simulink model "SiEnginePx"  (R2021b)
settings: Solver=VariableStepAuto  StartTime=0.0  StopTime=inf  RelTol=1e-3  EnableMultiTasking=on
InitFcn:
  | autoicon('autolibsiengcal',gcs,'varSwitched');
model workspace (MAT data in the model file):
  AccPwrbp = [0 0]
  AccSpdbp = [300 750]
  AfrStoich = 14.6
  TimeCnstECP = 0.125
  TimeCnstEGR = 0.125
  TimeCnstETC = 0.085
  TimeCnstICP = 0.125
  TimeCnstIVL = 0.125
  TimeCnstSWVA = 0.125
  TimeCnstVCR = 0.125
  TimeCnstVGT = 0.15
  TimeCnstVIRL = 0.125
  TimeCnstWGA = 0.15
  f_twc_eff_co = [0.17 0.25 0.45 0.99 0.99 0.99 0.99]
  f_twc_eff_hc = [0.21 0.375 0.75 0.98 0.98 0.98 0.98]
  f_twc_eff_lam = [0.909090909 0.944055944 0.979020979 1 1.013986014 1.048951049 1.083916084]
  f_twc_eff_nox = [0.98 0.98 0.98 0.97 0.05 0.02 0]
libraries: autolibhevctrlrcommon x1, autolibpowerinfoutils x1, autolibutils x1
settings Model: DataDictionary=SiEnginePx.sldd  ModifiedByFormat=The MathWorks, Inc.  SimulationMode=accelerator  Creator=The MathWorks, Inc.  LastModifiedBy=The MathWorks, Inc.
settings SolverCC: AlgebraicLoopSolver=TrustRegion  DecoupledContinuousIntegration=on
settings DataIOCC: DSMLogging=off  ReturnWorkspaceOutputs=off
settings DebuggingCC: ModelReferenceExtraNoncontSigs=none  SFMachineParentedDataDiag=warning  ArithmeticOperatorsInVariantConditions=warning
settings SFSimCC: SimUseLocalCustomCode=off  CustomCodeUndefinedFunction=UseInterfaceOnly
settings RTWCC: RTWUseLocalCustomCode=off
settings CodeAppCC: StateflowObjectComments=on
settings GRTTargetCC: TargetLangStandard=C89/C90 (ANSI)
settings ConfigComp: CovMetricSettings=dsw  CovSaveCumulativeToWorkspaceVar=on  CovSaveSingleToWorkspaceVar=on  CovExternalEMLEnable=off
settings SimscapeCC: SimscapeNormalizeSystem=off  SimscapeNominalValues={1, 'bar'; 1, 'cm^3/s'; 1, 'bar*kg/s'; 1, 'kJ/kg'; 1, 'kW'; };

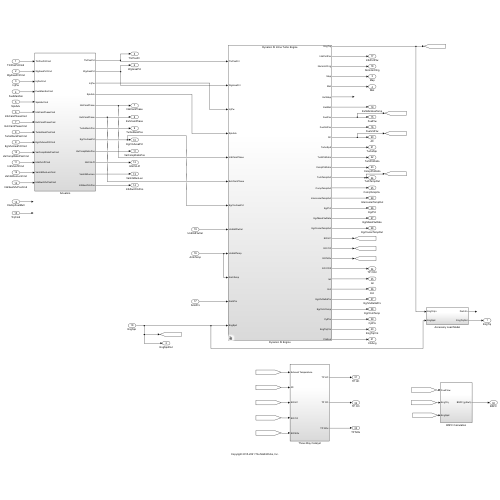
[thumbnail: Simulink's stored preview of the top-level diagram]
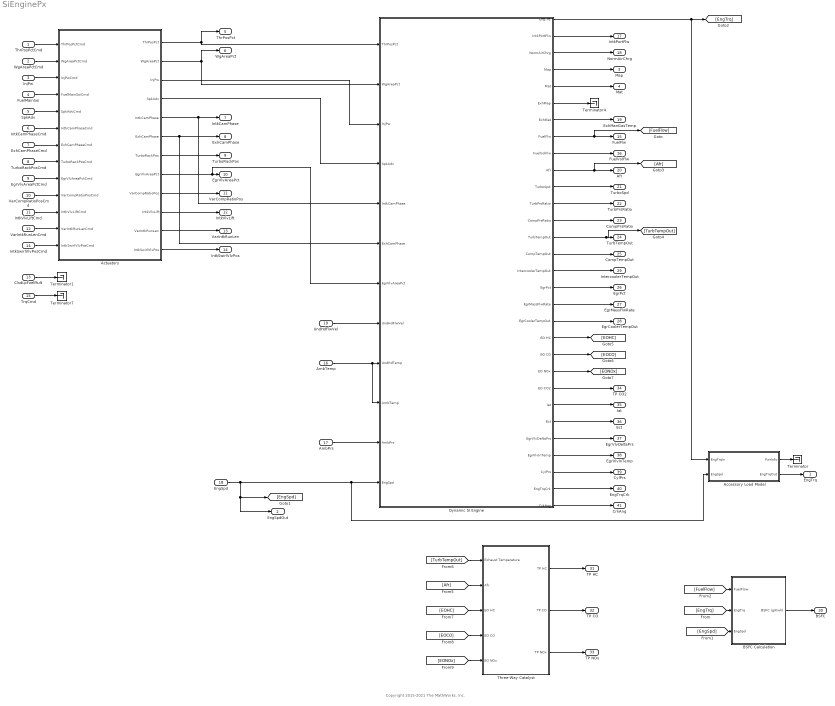
== system SiEnginePx ==
  note: Copyright 2015-2021 The MathWorks, Inc.
  ThrPosPctCmd : Inport
  WgAreaPctCmd : Inport  Port=2
  InjPw : Inport  Port=3
  FuelMainSoi : Inport  Port=4
  SpkAdv : Inport  Port=5
  IntkCamPhaseCmd : Inport  Port=6
  ExhCamPhaseCmd : Inport  Port=7
  TurboRackPosCmd : Inport  Port=8
  EgrVlvAreaPctCmd : Inport  Port=9
  VarCompRatioPosCmd : Inport  Port=10
  IntkVlvLiftCmd : Inport  Port=11
  VarIntkRunLenCmd : Inport  Port=12
  ClsdLpFuelMult : Inport  Port=13  Unit=1
  IntkSwirlVlvPosCmd : Inport  Port=14
  TrqCmd : Inport  Port=15  Unit=N*m
  AmbTemp : Inport  Port=16
  AmbPrs : Inport  Port=17
  EngSpd : Inport  Port=18  Interpolate=off
  UndHdFlwVel : Inport  Port=19
  Accessory Load Model : Subsystem
  Actuators : Subsystem
  BSFC Calculation : Subsystem
  Dynamic SI Engine : Subsystem  Variant=on  VariantControlMode=label  VariantControl=Choice  LabelModeActiveChoice=SiEngineCore
  Terminator{,1,4,7} (4 alike) : Terminator
  Three-Way Catalyst : Subsystem
  EngTrq : Outport  Unit=N*m  VectorParamsAs1DForOutWhenUnconnected=off
  EngSpdOut : Outport  Port=2  VectorParamsAs1DForOutWhenUnconnected=off
  Map : Outport  Port=3  VectorParamsAs1DForOutWhenUnconnected=off
  Mat : Outport  Port=4  VectorParamsAs1DForOutWhenUnconnected=off
  ThrPosPct : Outport  Port=5  VectorParamsAs1DForOutWhenUnconnected=off
  WgAreaPct : Outport  Port=6  VectorParamsAs1DForOutWhenUnconnected=off
  IntkCamPhase : Outport  Port=7  VectorParamsAs1DForOutWhenUnconnected=off
  ExhCamPhase : Outport  Port=8  VectorParamsAs1DForOutWhenUnconnected=off
  TurboRackPos : Outport  Port=9  VectorParamsAs1DForOutWhenUnconnected=off
  EgrVlvAreaPct : Outport  Port=10  VectorParamsAs1DForOutWhenUnconnected=off
  VarCompRatioPos : Outport  Port=11  VectorParamsAs1DForOutWhenUnconnected=off
  IntkVlvLift : Outport  Port=12  VectorParamsAs1DForOutWhenUnconnected=off
  VarIntkRunLen : Outport  Port=13  VectorParamsAs1DForOutWhenUnconnected=off
  IntkSwirlVlvPos : Outport  Port=14  VectorParamsAs1DForOutWhenUnconnected=off
  FuelFlw : Outport  Port=15  VectorParamsAs1DForOutWhenUnconnected=off
  FuelVolFlw : Outport  Port=16  VectorParamsAs1DForOutWhenUnconnected=off
  IntkPortFlw : Outport  Port=17  VectorParamsAs1DForOutWhenUnconnected=off
  NormAirChrg : Outport  Port=18  VectorParamsAs1DForOutWhenUnconnected=off
  ExhManGasTemp : Outport  Port=19  VectorParamsAs1DForOutWhenUnconnected=off
  Afr : Outport  Port=20  VectorParamsAs1DForOutWhenUnconnected=off
  TurboSpd : Outport  Port=21  VectorParamsAs1DForOutWhenUnconnected=off
  TurbPrsRatio : Outport  Port=22  VectorParamsAs1DForOutWhenUnconnected=off
  CompPrsRatio : Outport  Port=23  VectorParamsAs1DForOutWhenUnconnected=off
  TurbTempOut : Outport  Port=24  VectorParamsAs1DForOutWhenUnconnected=off
  CompTempOut : Outport  Port=25  VectorParamsAs1DForOutWhenUnconnected=off
  EgrPct : Outport  Port=26  Unit=%  VectorParamsAs1DForOutWhenUnconnected=off
  EgrMassFlwRate : Outport  Port=27  Unit=kg/s  VectorParamsAs1DForOutWhenUnconnected=off
  EgrCoolerTempOut : Outport  Port=28  Unit=K  VectorParamsAs1DForOutWhenUnconnected=off
  IntercoolerTempOut : Outport  Port=29  VectorParamsAs1DForOutWhenUnconnected=off
  BSFC : Outport  Port=30  Unit=g/(kW*hr)  VectorParamsAs1DForOutWhenUnconnected=off
  TP HC : Outport  Port=31  VectorParamsAs1DForOutWhenUnconnected=off
  TP CO : Outport  Port=32  VectorParamsAs1DForOutWhenUnconnected=off
  TP NOx : Outport  Port=33  VectorParamsAs1DForOutWhenUnconnected=off
  TP CO2 : Outport  Port=34  VectorParamsAs1DForOutWhenUnconnected=off
  Iat : Outport  Port=35  VectorParamsAs1DForOutWhenUnconnected=off
  Ect : Outport  Port=36  VectorParamsAs1DForOutWhenUnconnected=off
  EgrVlvDeltaPrs : Outport  Port=37  VectorParamsAs1DForOutWhenUnconnected=off
  EgrVlvInTemp : Outport  Port=38  VectorParamsAs1DForOutWhenUnconnected=off
  CylPrs : Outport  Port=39  VectorParamsAs1DForOutWhenUnconnected=off
  EngTrqCrk : Outport  Port=40  VectorParamsAs1DForOutWhenUnconnected=off
  CrkAng : Outport  Port=41  VectorParamsAs1DForOutWhenUnconnected=off
  wires:
  SpkAdv/1 -> Actuators/5(SpkAdvCmd)
  InjPw/1 -> Actuators/3(InjPwCmd)
  EngSpd/1 -> EngSpdOut/1, [EngSpd], Dynamic SI Engine/12(EngSpd), Accessory Load Model/2(EngSpd)
  [FuelFlow] -> BSFC Calculation/1(FuelFlow)
  [EngTrq] -> BSFC Calculation/2(EngTrq)
  [EngSpd] -> BSFC Calculation/3(EngSpd)
  BSFC Calculation/1(BSFC (g/Kwh)) -> BSFC/1
  Three-Way Catalyst/1(TP HC) -> TP HC/1
  Three-Way Catalyst/2(TP CO) -> TP CO/1
  Three-Way Catalyst/3(TP NOx) -> TP NOx/1
  [TurbTempOut] -> Three-Way Catalyst/1(Exhaust Temperature)
  [Afr] -> Three-Way Catalyst/2(Afr)
  ThrPosPctCmd/1 -> Actuators/1(ThrPosPctCmd)
  WgAreaPctCmd/1 -> Actuators/2(WgAreaPctCmd)
  IntkCamPhaseCmd/1 -> Actuators/6(IntkCamPhaseCmd)
  ExhCamPhaseCmd/1 -> Actuators/7(ExhCamPhaseCmd)
  TrqCmd/1 -> Terminator7/1
  [EOHC] -> Three-Way Catalyst/3(EO HC)
  [EOCO] -> Three-Way Catalyst/4(EO CO)
  [EONOx] -> Three-Way Catalyst/5(EO NOx)
  Actuators/1(ThrPosPct) -> ThrPosPct/1, Dynamic SI Engine/1(ThrPosPct)
  Actuators/2(WgAreaPct) -> WgAreaPct/1, Dynamic SI Engine/2(WgAreaPct)
  Actuators/5(IntkCamPhase) -> IntkCamPhase/1, Dynamic SI Engine/5(IntkCamPhase)
  Actuators/6(ExhCamPhase) -> ExhCamPhase/1, Dynamic SI Engine/6(ExhCamPhase)
  FuelMainSoi/1 -> Actuators/4(FuelMainSoiCmd)
  TurboRackPosCmd/1 -> Actuators/8(TurboRackPosCmd)
  EgrVlvAreaPctCmd/1 -> Actuators/9(EgrVlvAreaPctCmd)
  VarCompRatioPosCmd/1 -> Actuators/10(VarCompRatioPosCmd)
  IntkVlvLiftCmd/1 -> Actuators/11(IntkVlvLiftCmd)
  VarIntkRunLenCmd/1 -> Actuators/12(VarIntkRunLenCmd)
  IntkSwirlVlvPosCmd/1 -> Actuators/13(IntkSwirlVlvPosCmd)
  Actuators/7(TurboRackPos) -> TurboRackPos/1
  Actuators/8(EgrVlvAreaPct) -> EgrVlvAreaPct/1, Dynamic SI Engine/7(EgrVlvAreaPct)
  Actuators/9(VarCompRatioPos) -> VarCompRatioPos/1
  Actuators/10(IntkVlvLift) -> IntkVlvLift/1
  Actuators/11(VarIntkRunLen) -> VarIntkRunLen/1
  Actuators/12(IntkSwirlVlvPos) -> IntkSwirlVlvPos/1
  Accessory Load Model/2(EngTrqOut) -> EngTrq/1
  Accessory Load Model/1(PwrInfo) -> Terminator/1
  ClsdLpFuelMult/1 -> Terminator1/1
  Actuators/3(InjPw) -> Dynamic SI Engine/3(InjPw)
  Actuators/4(SpkAdv) -> Dynamic SI Engine/4(SpkAdv)
  UndHdFlwVel/1 -> Dynamic SI Engine/8(UndHdFlwVel)
  AmbTemp/1 -> Dynamic SI Engine/9(UndHdTemp), Dynamic SI Engine/10(AmbTemp)
  AmbPrs/1 -> Dynamic SI Engine/11(AmbPrs)
  Dynamic SI Engine/1(EngTrq) -> [EngTrq], Accessory Load Model/1(EngTrqIn)
  Dynamic SI Engine/2(IntkPortFlw) -> IntkPortFlw/1
  Dynamic SI Engine/3(NormAirChrg) -> NormAirChrg/1
  Dynamic SI Engine/4(Map) -> Map/1
  Dynamic SI Engine/5(Mat) -> Mat/1
  Dynamic SI Engine/6(ExhMap) -> Terminator4/1
  Dynamic SI Engine/7(ExhMat) -> ExhManGasTemp/1
  Dynamic SI Engine/8(FuelFlw) -> FuelFlw/1, [FuelFlow]
  Dynamic SI Engine/9(FuelVolFlw) -> FuelVolFlw/1
  Dynamic SI Engine/10(Afr) -> Afr/1, [Afr]
  Dynamic SI Engine/11(TurboSpd) -> TurboSpd/1
  Dynamic SI Engine/12(TurbPrsRatio) -> TurbPrsRatio/1
  Dynamic SI Engine/13(CompPrsRatio) -> CompPrsRatio/1
  Dynamic SI Engine/14(TurbTempOut) -> [TurbTempOut], TurbTempOut/1
  Dynamic SI Engine/15(CompTempOut) -> CompTempOut/1
  Dynamic SI Engine/16(IntercoolerTempOut) -> IntercoolerTempOut/1
  Dynamic SI Engine/17(EgrPct) -> EgrPct/1
  Dynamic SI Engine/18(EgrMassFlwRate) -> EgrMassFlwRate/1
  Dynamic SI Engine/19(EgrCoolerTempOut) -> EgrCoolerTempOut/1
  Dynamic SI Engine/20(EO HC) -> [EOHC]
  Dynamic SI Engine/21(EO CO) -> [EOCO]
  Dynamic SI Engine/22(EO NOx) -> [EONOx]
  Dynamic SI Engine/23(EO CO2) -> TP CO2/1
  Dynamic SI Engine/24(Iat) -> Iat/1
  Dynamic SI Engine/25(Ect) -> Ect/1
  Dynamic SI Engine/26(EgrVlvDeltaPrs) -> EgrVlvDeltaPrs/1
  Dynamic SI Engine/27(EgrVlvInTemp) -> EgrVlvInTemp/1
  Dynamic SI Engine/28(CylPrs) -> CylPrs/1
  Dynamic SI Engine/29(EngTrqCrk) -> EngTrqCrk/1
  Dynamic SI Engine/30(CrkAng) -> CrkAng/1

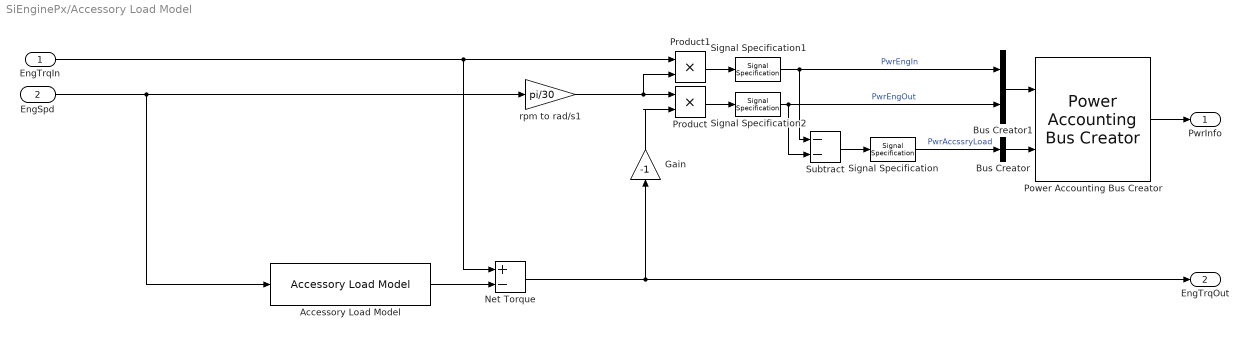
== system SiEnginePx/Accessory Load Model ==
  EngTrqIn : Inport
  EngSpd : Inport  Port=2
  Accessory Load Model : autolibhevctrlrcommon/Accessory Load Model  AccPwrTbl=[0 0]  AccSpdBpts=[300 750]
      settings: SourceProductBaseCode=PW
  Bus Creator : BusCreator  Inputs=1
  Bus Creator1 : BusCreator  Inputs=2
  Gain : Gain  Gain=-1
  Net Torque : Sum  Inputs=+-
  Power Accounting Bus Creator : autolibpowerinfoutils/Power Accounting Bus Creator  AssctBlkSelPopup=Parent  RefBlkName='libraryname/blkname'  PwrTrnsfrdCheckBox=on  PwrNotTrnsfrdCheckBox=on  PwrStoredCheckBox=off  aMode=aMode
      settings: SourceProductBaseCode=PW,DR,MT,UV,VE
  Product : Product
  Product1 : Product
  Signal Specification : SignalSpecification  Unit=W
  Signal Specification1 : SignalSpecification  Unit=W
  Signal Specification2 : SignalSpecification  Unit=W
  Subtract : Sum  Inputs=--
  rpm to rad/s1 : Gain  Gain=pi/30
  PwrInfo : Outport  VectorParamsAs1DForOutWhenUnconnected=off
  EngTrqOut : Outport  Port=2  Unit=N*m  VectorParamsAs1DForOutWhenUnconnected=off
  wires:
  Accessory Load Model/1 -> Net Torque/2
  EngSpd/1 -> Accessory Load Model/1, rpm to rad/s1/1
  Net Torque/1 -> EngTrqOut/1, Gain/1
  Bus Creator/1 -> Power Accounting Bus Creator/2
  Bus Creator1/1 -> Power Accounting Bus Creator/1
  EngTrqIn/1 -> Product1/1, Net Torque/1
  Subtract/1 -> Signal Specification/1
  Signal Specification/1 -> Bus Creator/1  "PwrAccssryLoad"
  Power Accounting Bus Creator/1 -> PwrInfo/1
  Product/1 -> Signal Specification2/1
  Product1/1 -> Signal Specification1/1
  rpm to rad/s1/1 -> Product1/2, Product/1
  Signal Specification1/1 -> Subtract/1, Bus Creator1/1  "PwrEngIn"
  Signal Specification2/1 -> Subtract/2, Bus Creator1/2  "PwrEngOut"
  Gain/1 -> Product/2

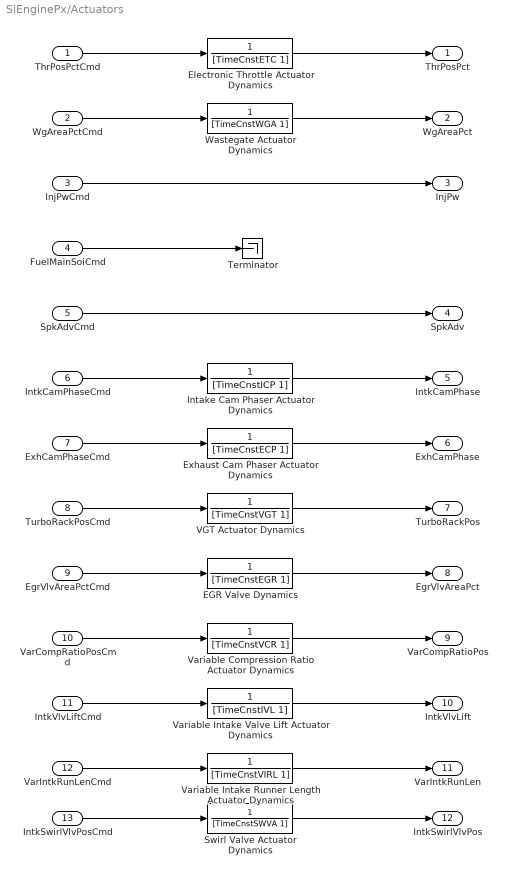
== system SiEnginePx/Actuators ==
  ThrPosPctCmd : Inport  Unit=%
  WgAreaPctCmd : Inport  Port=2  Unit=%
  InjPwCmd : Inport  Port=3  Unit=ms
  FuelMainSoiCmd : Inport  Port=4  Unit=deg
  SpkAdvCmd : Inport  Port=5  Unit=deg
  IntkCamPhaseCmd : Inport  Port=6  Unit=deg
  ExhCamPhaseCmd : Inport  Port=7  Unit=deg
  TurboRackPosCmd : Inport  Port=8  Unit=1
  EgrVlvAreaPctCmd : Inport  Port=9  Unit=%
  VarCompRatioPosCmd : Inport  Port=10
  IntkVlvLiftCmd : Inport  Port=11
  VarIntkRunLenCmd : Inport  Port=12
  IntkSwirlVlvPosCmd : Inport  Port=13
  EGR Valve Dynamics : TransferFcn  Denominator=[TimeCnstEGR 1]
  Electronic Throttle Actuator Dynamics : TransferFcn  Denominator=[TimeCnstETC 1]
  Exhaust Cam Phaser Actuator Dynamics : TransferFcn  Denominator=[TimeCnstECP 1]
  Intake Cam Phaser Actuator Dynamics : TransferFcn  Denominator=[TimeCnstICP 1]
  Swirl Valve Actuator Dynamics : TransferFcn  Denominator=[TimeCnstSWVA 1]
  Terminator : Terminator
  VGT Actuator Dynamics : TransferFcn  Denominator=[TimeCnstVGT 1]
  Variable Compression Ratio Actuator Dynamics : TransferFcn  Denominator=[TimeCnstVCR 1]
  Variable Intake Runner Length Actuator Dynamics : TransferFcn  Denominator=[TimeCnstVIRL 1]
  Variable Intake Valve Lift Actuator Dynamics : TransferFcn  Denominator=[TimeCnstIVL 1]
  Wastegate Actuator Dynamics : TransferFcn  Denominator=[TimeCnstWGA 1]
  ThrPosPct : Outport  Unit=%  VectorParamsAs1DForOutWhenUnconnected=off
  WgAreaPct : Outport  Port=2  Unit=%  VectorParamsAs1DForOutWhenUnconnected=off
  InjPw : Outport  Port=3  VectorParamsAs1DForOutWhenUnconnected=off
  SpkAdv : Outport  Port=4  VectorParamsAs1DForOutWhenUnconnected=off
  IntkCamPhase : Outport  Port=5  Unit=deg  VectorParamsAs1DForOutWhenUnconnected=off
  ExhCamPhase : Outport  Port=6  Unit=deg  VectorParamsAs1DForOutWhenUnconnected=off
  TurboRackPos : Outport  Port=7  Unit=1  VectorParamsAs1DForOutWhenUnconnected=off
  EgrVlvAreaPct : Outport  Port=8  Unit=%  VectorParamsAs1DForOutWhenUnconnected=off
  VarCompRatioPos : Outport  Port=9  VectorParamsAs1DForOutWhenUnconnected=off
  IntkVlvLift : Outport  Port=10  VectorParamsAs1DForOutWhenUnconnected=off
  VarIntkRunLen : Outport  Port=11  VectorParamsAs1DForOutWhenUnconnected=off
  IntkSwirlVlvPos : Outport  Port=12  VectorParamsAs1DForOutWhenUnconnected=off
  wires:
  Variable Compression Ratio Actuator Dynamics/1 -> VarCompRatioPos/1
  Variable Intake Valve Lift Actuator Dynamics/1 -> IntkVlvLift/1
  Variable Intake Runner Length Actuator Dynamics/1 -> VarIntkRunLen/1
  Swirl Valve Actuator Dynamics/1 -> IntkSwirlVlvPos/1
  Intake Cam Phaser Actuator Dynamics/1 -> IntkCamPhase/1
  Exhaust Cam Phaser Actuator Dynamics/1 -> ExhCamPhase/1
  Wastegate Actuator Dynamics/1 -> WgAreaPct/1
  Electronic Throttle Actuator Dynamics/1 -> ThrPosPct/1
  FuelMainSoiCmd/1 -> Terminator/1
  IntkVlvLiftCmd/1 -> Variable Intake Valve Lift Actuator Dynamics/1
  IntkSwirlVlvPosCmd/1 -> Swirl Valve Actuator Dynamics/1
  WgAreaPctCmd/1 -> Wastegate Actuator Dynamics/1
  ThrPosPctCmd/1 -> Electronic Throttle Actuator Dynamics/1
  ExhCamPhaseCmd/1 -> Exhaust Cam Phaser Actuator Dynamics/1
  IntkCamPhaseCmd/1 -> Intake Cam Phaser Actuator Dynamics/1
  VarCompRatioPosCmd/1 -> Variable Compression Ratio Actuator Dynamics/1
  VarIntkRunLenCmd/1 -> Variable Intake Runner Length Actuator Dynamics/1
  InjPwCmd/1 -> InjPw/1
  VGT Actuator Dynamics/1 -> TurboRackPos/1
  EGR Valve Dynamics/1 -> EgrVlvAreaPct/1
  TurboRackPosCmd/1 -> VGT Actuator Dynamics/1
  EgrVlvAreaPctCmd/1 -> EGR Valve Dynamics/1
  SpkAdvCmd/1 -> SpkAdv/1

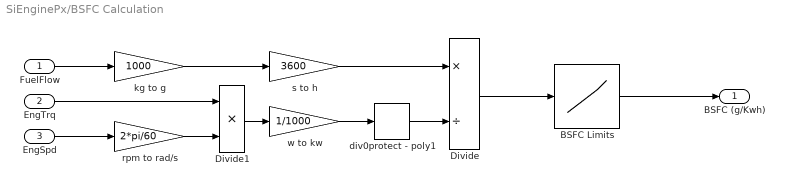
== system SiEnginePx/BSFC Calculation ==
  FuelFlow : Inport
  EngTrq : Inport  Port=2
  EngSpd : Inport  Port=3
  BSFC Limits : Lookup_n-D  NumberOfTableDimensions=1  BreakpointsForDimension1=[0 500]  Table=[0 500]  ExtrapMethod=Clip  InternalRulePriority=Speed  RndMeth=Simplest  InputSameDT=on
  Divide : Product  Inputs=*/
  Divide1 : Product  Inputs=**
  div0protect - poly1 : autolibutils/div0protect - poly  thresh=1e-6  ZeroCross1=off  aMode=aMode
      settings: SourceProductBaseCode=PW,DR,MT,UV,VE
  kg to g : Gain  Gain=1000
  rpm to rad/s : Gain  Gain=2*pi/60
  s to h : Gain  Gain=3600
  w to kw : Gain  Gain=1/1000
  BSFC (g/Kwh) : Outport  VectorParamsAs1DForOutWhenUnconnected=off
  wires:
  Divide1/1 -> w to kw/1
  kg to g/1 -> s to h/1
  FuelFlow/1 -> kg to g/1
  rpm to rad/s/1 -> Divide1/2
  EngSpd/1 -> rpm to rad/s/1
  EngTrq/1 -> Divide1/1
  Divide/1 -> BSFC Limits/1
  w to kw/1 -> div0protect - poly1/1
  s to h/1 -> Divide/1
  BSFC Limits/1 -> BSFC (g/Kwh)/1
  div0protect - poly1/1 -> Divide/2

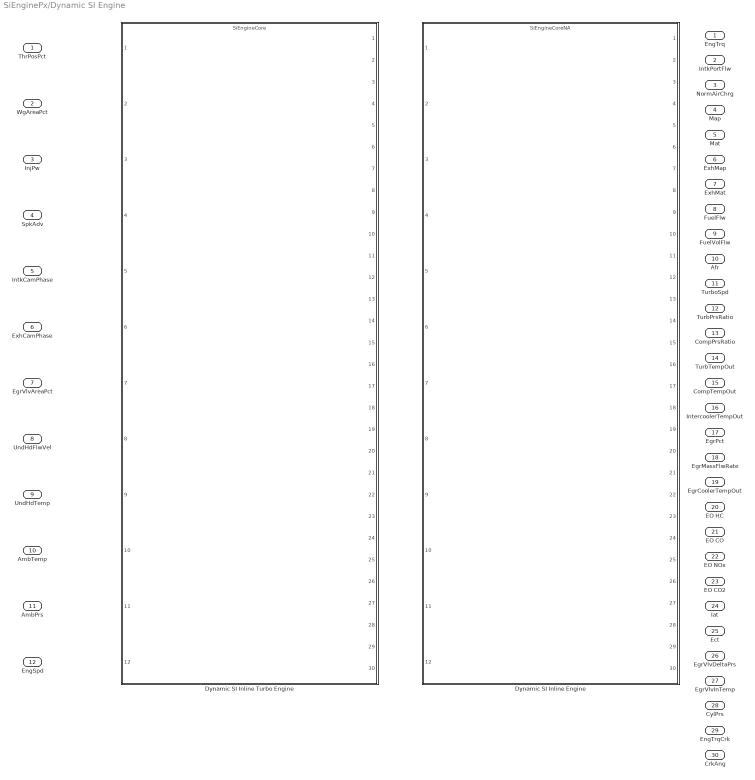
== system SiEnginePx/Dynamic SI Engine ==
  ThrPosPct : Inport
  WgAreaPct : Inport  Port=2
  InjPw : Inport  Port=3
  SpkAdv : Inport  Port=4
  IntkCamPhase : Inport  Port=5
  ExhCamPhase : Inport  Port=6
  EgrVlvAreaPct : Inport  Port=7
  UndHdFlwVel : Inport  Port=8
  UndHdTemp : Inport  Port=9
  AmbTemp : Inport  Port=10
  AmbPrs : Inport  Port=11
  EngSpd : Inport  Port=12
  Dynamic SI Inline Engine : ModelReference  ModelNameDialog=SiEngineCoreNA.slx  SimulationMode=Normal  VariantControl=SiEngineCoreNA  ModelReferenceVersion=3.4
  Dynamic SI Inline Turbo Engine : ModelReference  ModelNameDialog=SiEngineCore.slx  SimulationMode=Normal  VariantControl=SiEngineCore  ModelReferenceVersion=3.4
  EngTrq : Outport
  IntkPortFlw : Outport  Port=2
  NormAirChrg : Outport  Port=3
  Map : Outport  Port=4
  Mat : Outport  Port=5
  ExhMap : Outport  Port=6
  ExhMat : Outport  Port=7
  FuelFlw : Outport  Port=8
  FuelVolFlw : Outport  Port=9
  Afr : Outport  Port=10
  TurboSpd : Outport  Port=11
  TurbPrsRatio : Outport  Port=12
  CompPrsRatio : Outport  Port=13
  TurbTempOut : Outport  Port=14
  CompTempOut : Outport  Port=15
  IntercoolerTempOut : Outport  Port=16
  EgrPct : Outport  Port=17
  EgrMassFlwRate : Outport  Port=18
  EgrCoolerTempOut : Outport  Port=19
  EO HC : Outport  Port=20
  EO CO : Outport  Port=21
  EO NOx : Outport  Port=22
  EO CO2 : Outport  Port=23
  Iat : Outport  Port=24
  Ect : Outport  Port=25
  EgrVlvDeltaPrs : Outport  Port=26
  EgrVlvInTemp : Outport  Port=27
  CylPrs : Outport  Port=28  VectorParamsAs1DForOutWhenUnconnected=off
  EngTrqCrk : Outport  Port=29  VectorParamsAs1DForOutWhenUnconnected=off
  CrkAng : Outport  Port=30  VectorParamsAs1DForOutWhenUnconnected=off

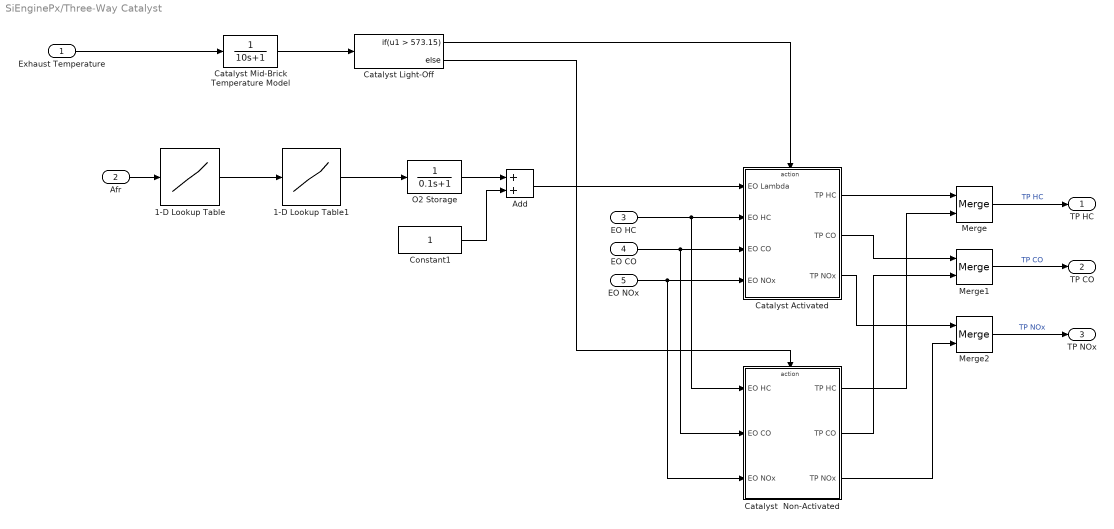
== system SiEnginePx/Three-Way Catalyst ==
  Exhaust Temperature : Inport
  Afr : Inport  Port=2
  EO HC : Inport  Port=3
  EO CO : Inport  Port=4
  EO NOx : Inport  Port=5
  1-D Lookup Table : Lookup_n-D  NumberOfTableDimensions=1  BreakpointsForDimension1=[0 15 100]  Table=[0 15 AfrStoich]/AfrStoich  ExtrapMethod=Clip  InternalRulePriority=Speed  RndMeth=Simplest  InputSameDT=on
  1-D Lookup Table1 : Lookup_n-D  NumberOfTableDimensions=1  BreakpointsForDimension1=[0 0.97 1.03 1.1]  Table=[-1 0 0 0.07]  ExtrapMethod=Clip  InternalRulePriority=Speed  RndMeth=Simplest  InputSameDT=on
  Add : Sum
  Catalyst  Non-Activated : Subsystem
  Catalyst Activated : Subsystem
  Catalyst Light-Off : If  IfExpression=u1 > 573.15
  "Catalyst Mid-Brick Temperature Model " : TransferFcn  Denominator=[10 1]
  Constant1 : Constant
  Merge : Merge
  Merge1 : Merge
  Merge2 : Merge
  O2 Storage : TransferFcn  Denominator=[0.1 1]
  TP HC : Outport  Unit=kg/s  VectorParamsAs1DForOutWhenUnconnected=off
  TP CO : Outport  Port=2  Unit=kg/s  VectorParamsAs1DForOutWhenUnconnected=off
  TP NOx : Outport  Port=3  Unit=kg/s  VectorParamsAs1DForOutWhenUnconnected=off
  wires:
  EO HC/1 -> Catalyst  Non-Activated/1(EO HC), Catalyst Activated/2(EO HC)
  EO CO/1 -> Catalyst  Non-Activated/2(EO CO), Catalyst Activated/3(EO CO)
  EO NOx/1 -> Catalyst  Non-Activated/3(EO NOx), Catalyst Activated/4(EO NOx)
  Merge/1 -> TP HC/1  "TP HC"
  Merge1/1 -> TP CO/1  "TP CO"
  Merge2/1 -> TP NOx/1  "TP NOx"
  Exhaust Temperature/1 -> "Catalyst Mid-Brick Temperature Model "/1
  Catalyst Light-Off/1 -> Catalyst Activated/Action
  Catalyst Light-Off/2 -> Catalyst  Non-Activated/Action
  "Catalyst Mid-Brick Temperature Model "/1 -> Catalyst Light-Off/1
  Catalyst Activated/1(TP HC) -> Merge/1
  Catalyst  Non-Activated/1(TP HC) -> Merge/2
  Catalyst Activated/2(TP CO) -> Merge1/1
  Catalyst  Non-Activated/2(TP CO) -> Merge1/2
  Catalyst Activated/3(TP NOx) -> Merge2/1
  Catalyst  Non-Activated/3(TP NOx) -> Merge2/2
  Add/1 -> Catalyst Activated/1(EO Lambda)
  1-D Lookup Table1/1 -> O2 Storage/1
  Constant1/1 -> Add/2
  O2 Storage/1 -> Add/1
  Afr/1 -> 1-D Lookup Table/1
  1-D Lookup Table/1 -> 1-D Lookup Table1/1

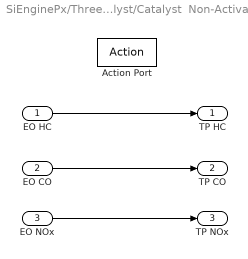
== system SiEnginePx/Three-Way Catalyst/Catalyst  Non-Activated ==
  EO HC : Inport
  EO CO : Inport  Port=2
  EO NOx : Inport  Port=3
  Action Port : ActionPort  ActionPortLabel=else
  TP HC : Outport  VectorParamsAs1DForOutWhenUnconnected=off
  TP CO : Outport  Port=2  VectorParamsAs1DForOutWhenUnconnected=off
  TP NOx : Outport  Port=3  VectorParamsAs1DForOutWhenUnconnected=off
  wires:
  EO HC/1 -> TP HC/1
  EO CO/1 -> TP CO/1
  EO NOx/1 -> TP NOx/1

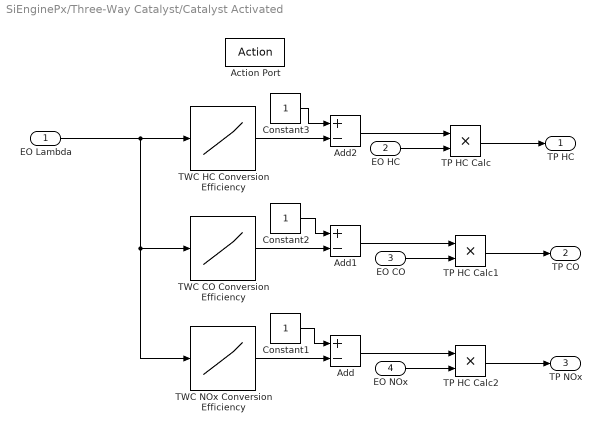
== system SiEnginePx/Three-Way Catalyst/Catalyst Activated ==
  EO Lambda : Inport
  EO HC : Inport  Port=2
  EO CO : Inport  Port=3
  EO NOx : Inport  Port=4
  Action Port : ActionPort  ActionPortLabel=if(u1 > 573.15)
  Add : Sum  Inputs=+-
  Add1 : Sum  Inputs=+-
  Add2 : Sum  Inputs=+-
  Constant1 : Constant
  Constant2 : Constant
  Constant3 : Constant
  TP HC Calc : Product  Inputs=**
  TP HC Calc1 : Product  Inputs=**
  TP HC Calc2 : Product  Inputs=**
  TWC CO Conversion Efficiency : Lookup_n-D  NumberOfTableDimensions=1  LookupTableObject=''  BreakpointsForDimension1=f_twc_eff_lam  Table=f_twc_eff_co  ExtrapMethod=Clip  InternalRulePriority=Speed  RndMeth=Simplest  InputSameDT=on
  TWC HC Conversion Efficiency : Lookup_n-D  NumberOfTableDimensions=1  LookupTableObject=''  BreakpointsForDimension1=f_twc_eff_lam  Table=f_twc_eff_hc  ExtrapMethod=Clip  InternalRulePriority=Speed  RndMeth=Simplest  InputSameDT=on
  TWC NOx Conversion Efficiency : Lookup_n-D  NumberOfTableDimensions=1  LookupTableObject=''  BreakpointsForDimension1=f_twc_eff_lam  Table=f_twc_eff_nox  ExtrapMethod=Clip  InternalRulePriority=Speed  RndMeth=Simplest  InputSameDT=on
  TP HC : Outport  VectorParamsAs1DForOutWhenUnconnected=off
  TP CO : Outport  Port=2  VectorParamsAs1DForOutWhenUnconnected=off
  TP NOx : Outport  Port=3  VectorParamsAs1DForOutWhenUnconnected=off
  wires:
  EO HC/1 -> TP HC Calc/2
  TP HC Calc/1 -> TP HC/1
  Add/1 -> TP HC Calc2/1
  Constant1/1 -> Add/1
  TP HC Calc1/1 -> TP CO/1
  TWC HC Conversion Efficiency/1 -> Add2/2
  Add1/1 -> TP HC Calc1/1
  EO CO/1 -> TP HC Calc1/2
  TP HC Calc2/1 -> TP NOx/1
  EO NOx/1 -> TP HC Calc2/2
  EO Lambda/1 -> TWC NOx Conversion Efficiency/1, TWC CO Conversion Efficiency/1, TWC HC Conversion Efficiency/1
  Constant2/1 -> Add1/1
  TWC CO Conversion Efficiency/1 -> Add1/2
  Constant3/1 -> Add2/1
  Add2/1 -> TP HC Calc/1
  TWC NOx Conversion Efficiency/1 -> Add/2
